simulink model "test_only"  (R2020a)
settings: Solver=FixedStepDiscrete  StartTime=0.0  StopTime=Parm_cnv_simulink_stopTime  FixedStep=Const_cnv_fundmt_stepSize  RelTol=1e-3  EnableMultiTasking=on
InitFcn:
  | preLoadFun
libraries: speedgoatlib_IO691 x9, canmsglib x9, MyLibrary x1, libtb_gen_canMsgCntr x1
Description:
  | - Add preLoadFun.m into Callbacks InitFcn
  | - Combine Sensata and Pirelle sensor inputs into one subsystem
  | - Two enumerators: defEnum_fun_tbm.m && def_vehFun_Enum.m
settings Model: SimulationMode=external  PauseTimes=49.73  NumberOfSteps=20  EnablePacing=on  PacingRate=112  Creator=jianjun.gao  LastModifiedBy=bowen.zheng
settings SolverCC: ConcurrentTasks=on  AlgebraicLoopSolver=LineSearch  AutoInsertRateTranBlk=on
settings DataIOCC: LimitDataPoints=on  SaveFormat=StructureWithTime  ReturnWorkspaceOutputs=off
settings OptimizationCC: BlockReduction=off  DefaultUnderspecifiedDataType=single  OptimizeBlockIOStorage=off  EnhancedBackFolding=on  PassReuseOutputArgsThreshold=0  ExpressionDepthLimit=2147483647  OptimizeBlockOrder=speed  DifferentSizesBufferReuse=on
settings DebuggingCC: UnderspecifiedInitializationDetection=Classic  MergeDetectMultiDrivingBlocksExec=none  SolverPrmCheckMsg=warning  ParameterTunabilityLossMsg=error  FcnCallInpInsideContextMsg=warning  BusObjectLabelMismatch=error  AllowSymbolicDim=off  StateNameClashWarn=warning  SFUnexpectedBacktrackingDiag=warning  SFNoUnconditionalDefaultTransitionDiag=warning  SFExecutionAtInitializationDiag=none  ArithmeticOperatorsInVariantConditions=warning
settings HardwareCC: ProdBitPerPointer=32  ProdBitPerSizeT=32  ProdBitPerPtrDiffT=32  ProdLargestAtomicFloat=None  ProdWordSize=32  ProdLongLongMode=on  ProdHWDeviceType=Generic->32-bit x86 compatible
settings ModelReferenceCC: PropagateSignalLabelsOutOfModel=off
settings SFSimCC: SimUseLocalCustomCode=off  MATLABDynamicMemAlloc=off  CustomCodeUndefinedFunction=UseInterfaceOnly
settings RTWCC: Description=Simulink Real-Time  SystemTargetFile=slrt.tlc  PackageName=addn_compled  TemplateMakefile=slrt_default_tmf  RTWUseLocalCustomCode=off  RTWUseSimCustomCode=on  BuildConfiguration=Faster Runs  CodeExecutionProfiling=on  RTWCompilerOptimization=on
settings CodeAppCC: ForceParamTrailComments=on  MaxIdLength=63  OperatorAnnotations=on
settings SimulinkRealTimeCC: SupportVariableSizeSignals=on  RL32LogTETModifier=off  xPCConcurrentTasks=on
settings ConfigComp: CovMetricSettings=dw  CovHtmlReporting=on  CovSaveCumulativeToWorkspaceVar=on  CovSaveSingleToWorkspaceVar=on  CovExternalEMLEnable=off
settings SimscapeCC: SimscapeNormalizeSystem=off
settings ConfigurationSet: Description=SimMechanics 2G

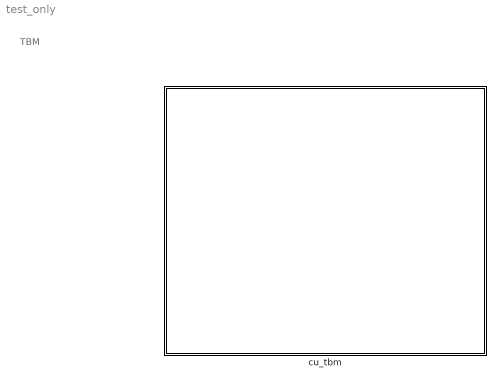
== system test_only ==
  note: TBM
  cu_tbm : Subsystem

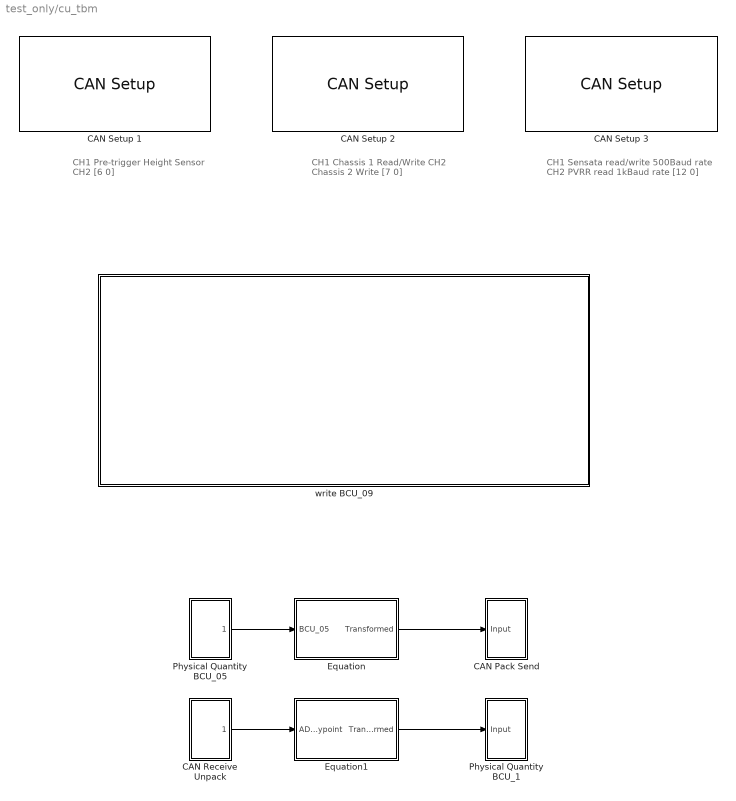
== system test_only/cu_tbm ==
  note: CH1 Pre-trigger Height Sensor
      | CH2
      | [6 0]
  note: CH1 Chassis 1 Read/Write
      | CH2 Chassis 2 Write
      | [7 0]
  note: CH1 Sensata read/write 500Baud rate
      | CH2 PVRR read 1kBaud rate
      | [12 0]
  CAN Pack Send : Subsystem
  CAN Receive Unpack : Subsystem
  CAN Setup 1 : speedgoatlib_IO691/CAN Setup   moduletype=IO691  id=1  pciSlot=[6 0]  chn1=CAN (HS)  chn2=CAN (HS)  chn3=Disabled  chn4=Disabled  initStruct=[]  termStruct=[]  ArbitrationbdrChn1=500 kBaud  ArbitrationManbdrChn1=[2,16,63,16]  FdbdrChn1=5.0 MBaud  FdManbdrChn1=[2,2,5,2]  ArbitrationbdrChn2=500 kBaud  ArbitrationManbdrChn2=[2,16,63,16]  FdbdrChn2=5.0 MBaud  FdManbdrChn2=[2,2,5,2]  ArbitrationbdrChn3=1.0 MBaud  ArbitrationManbdrChn3=[2,8,31,8]  FdbdrChn3=5.0 MBaud  FdManbdrChn3=[2,2,5,2]  ArbitrationbdrChn4=1.0 MBaud  ArbitrationManbdrChn4=[2,8,31,8]  FdbdrChn4=5.0 MBaud  FdManbdrChn4=[2,2,5,2]  moduleInitValues=[691 1 6 0]
      settings: SourceProductName=Simulink Real-Time: Speedgoat I/O Blockset
  CAN Setup 2 : speedgoatlib_IO691/CAN Setup   moduletype=IO691  id=2  pciSlot=[7 0]  chn1=CAN (HS)  chn2=CAN (HS)  chn3=Disabled  chn4=Disabled  initStruct=[]  termStruct=[]  ArbitrationbdrChn1=500 kBaud  ArbitrationManbdrChn1=[2,16,63,16]  FdbdrChn1=5.0 MBaud  FdManbdrChn1=[2,2,5,2]  ArbitrationbdrChn2=500 kBaud  ArbitrationManbdrChn2=[2,16,63,16]  FdbdrChn2=5.0 MBaud  FdManbdrChn2=[2,2,5,2]  ArbitrationbdrChn3=1.0 MBaud  ArbitrationManbdrChn3=[2,8,31,8]  FdbdrChn3=5.0 MBaud  FdManbdrChn3=[2,2,5,2]  ArbitrationbdrChn4=1.0 MBaud  ArbitrationManbdrChn4=[2,8,31,8]  FdbdrChn4=5.0 MBaud  FdManbdrChn4=[2,2,5,2]  moduleInitValues=[691 2 7 0]
      settings: SourceProductName=Simulink Real-Time: Speedgoat I/O Blockset
  CAN Setup 3 : speedgoatlib_IO691/CAN Setup   moduletype=IO691  id=4  pciSlot=[12 0]  chn1=CAN (HS)  chn2=CAN (HS)  chn3=Disabled  chn4=Disabled  initStruct=[]  termStruct=[]  ArbitrationbdrChn1=500 kBaud  ArbitrationManbdrChn1=[2,16,63,16]  FdbdrChn1=5.0 MBaud  FdManbdrChn1=[2,2,5,2]  ArbitrationbdrChn2=1.0 MBaud  ArbitrationManbdrChn2=[2,8,31,8]  FdbdrChn2=5.0 MBaud  FdManbdrChn2=[2,2,5,2]  ArbitrationbdrChn3=1.0 MBaud  ArbitrationManbdrChn3=[2,8,31,8]  FdbdrChn3=5.0 MBaud  FdManbdrChn3=[2,2,5,2]  ArbitrationbdrChn4=1.0 MBaud  ArbitrationManbdrChn4=[2,8,31,8]  FdbdrChn4=5.0 MBaud  FdManbdrChn4=[2,2,5,2]  moduleInitValues=[691 4 12 0]
      settings: SourceProductName=Simulink Real-Time: Speedgoat I/O Blockset
  Equation : Subsystem
  Equation1 : Subsystem
  Physical Quantity BCU_05 : Subsystem
  Physical Quantity BCU_1 : Subsystem
  write BCU_09 : Subsystem
  wires:
  Physical Quantity BCU_05/1(BCU_05) -> Equation/1(BCU_05)
  CAN Receive Unpack/1(Output) -> Equation1/1(ADC_Waypoint)
  Equation1/1(Transformed) -> Physical Quantity BCU_1/1(Input)
  Equation/1(Transformed) -> CAN Pack Send/1(Input)

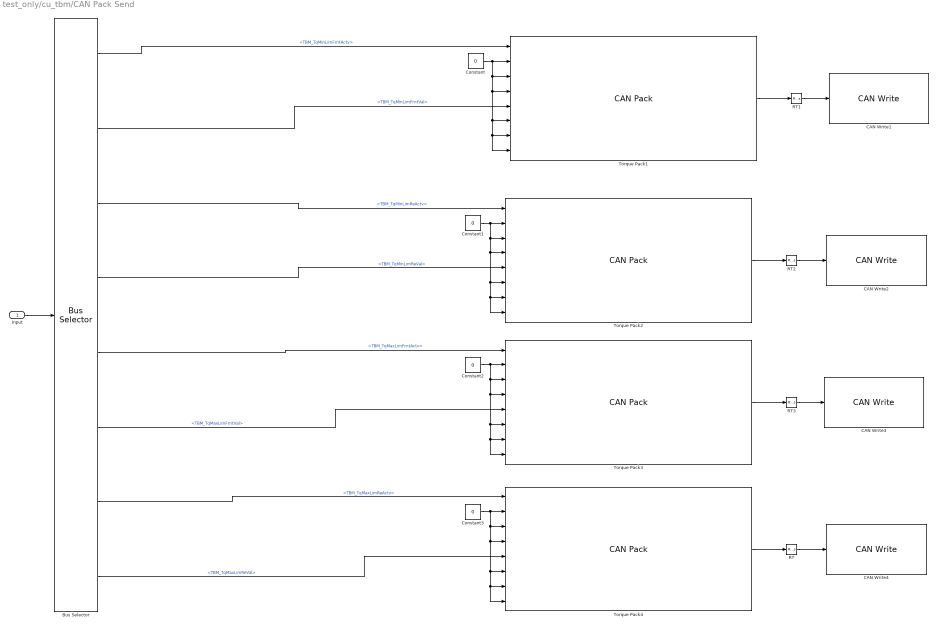
== system test_only/cu_tbm/CAN Pack Send ==
  Input : Inport
  Bus Selector : BusSelector  OutputSignals=TBM_TqMinLimFrntActv,TBM_TqMinLimFrntVal,TBM_TqMinLimReActv,TBM_TqMinLimReVal,TBM_TqMaxLimFrntActv,TBM_TqMaxLimFrntVal,TBM_TqMaxLimReActv,TBM_TqMaxLimReVal
  CAN Write{1..4} (4 alike) : speedgoatlib_IO691/CAN Write  id=2  ts=0.02  channel=1  messageType=CAN  enableStatusPort=off  canType=CAN (HS)  initValues=[691 2 0.02 0 1 1 0]
      settings: SourceProductName=Simulink Real-Time: Speedgoat I/O Blockset
  Constant{,1..3} (4 alike) : Constant  Value=0  OutDataTypeStr=single
  RT{,1..3} (4 alike) : RateTransition  OutPortSampleTime=0.02
  Torque Pack1 : canmsglib/CAN Pack  CANdbFile=.\support\dbc\NIO_NT2_Chassis2_CAN_Official_Release_V_1_1_DA_02.dbc  MsgList=ADC1_WayPoint01  MsgName=ADC1_WayPoint01  MsgIDType=Standard (11-bit identifier)  MsgIdentifier=214  MsgLength=8  Remote=off  ApplyMinMax=off  BusOutput=off  SignalInfo={'LD_Confidence_1','24','4','BE','unsigned','Standard','0','0.1','0','0','1.5';'LD_First_End_1','51','7','BE','unsigned','Standard','0','1','0','0','127';'LD_First_Start_1','16','8','BE','unsigned','Standard','0','0.1','0','0','25.5';'LD_First_Type_1','28','4','BE','unsigned','Standard','0','1','0','0','15';'LD_Line_First_C0_1','56','11','BE','unsigned','Standard','0','0.01','-10.24','-10.24','10.23';'LD_Line_First_C1_1','43','13','BE','unsigned','Standard','0','0.0001','-0.4096','-0.4096','0.4095';'LD_Line_First_C2_1','0','8','BE','unsigned','Standard','0','0.0001','-0.0128','-0.0128','0.0127';'LD_Line_First_C3_1','8','8','BE','unsigned','Standard','0','1e-06','-0.000128','-0.000128','0.000127'}
      settings: SourceProductBaseCode=ME,VN  DataFormat=CANdb specified signals
  Torque Pack2 : canmsglib/CAN Pack  CANdbFile=.\support\dbc\NIO_NT2_Chassis2_CAN_Official_Release_V_1_1_DA_02.dbc  MsgList=ADC1_WayPoint02  MsgName=ADC1_WayPoint02  MsgIDType=Standard (11-bit identifier)  MsgIdentifier=215  MsgLength=8  Remote=off  ApplyMinMax=off  BusOutput=off  SignalInfo={'LD_Confidence_2','24','4','BE','unsigned','Standard','0','0.1','0','0','1.5';'LD_First_End_2','51','7','BE','unsigned','Standard','0','1','0','0','127';'LD_First_Start_2','16','8','BE','unsigned','Standard','0','0.1','0','0','25.5';'LD_First_Type_2','28','4','BE','unsigned','Standard','0','1','0','0','15';'LD_Line_First_C0_2','56','11','BE','unsigned','Standard','0','0.01','-10.24','-10.24','10.23';'LD_Line_First_C1_2','43','13','BE','unsigned','Standard','0','0.0001','-0.4096','-0.4096','0.4095';'LD_Line_First_C2_2','0','8','BE','unsigned','Standard','0','0.0001','-0.0128','-0.0128','0.0127';'LD_Line_First_C3_2','8','8','BE','unsigned','Standard','0','1e-06','-0.000128','-0.000128','0.000127'}
      settings: SourceProductBaseCode=ME,VN  DataFormat=CANdb specified signals
  Torque Pack3 : canmsglib/CAN Pack  CANdbFile=.\support\dbc\NIO_NT2_Chassis2_CAN_Official_Release_V_1_1_DA_02.dbc  MsgList=ADC1_WayPoint03  MsgName=ADC1_WayPoint03  MsgIDType=Standard (11-bit identifier)  MsgIdentifier=216  MsgLength=8  Remote=off  ApplyMinMax=off  BusOutput=off  SignalInfo={'LD_Confidence_3','24','4','BE','unsigned','Standard','0','0.1','0','0','1.5';'LD_First_End_3','51','7','BE','unsigned','Standard','0','1','0','0','127';'LD_First_Start_3','16','8','BE','unsigned','Standard','0','0.1','0','0','25.5';'LD_First_Type_3','28','4','BE','unsigned','Standard','0','1','0','0','15';'LD_Line_First_C0_3','56','11','BE','unsigned','Standard','0','0.01','-10.24','-10.24','10.23';'LD_Line_First_C1_3','43','13','BE','unsigned','Standard','0','0.0001','-0.4096','-0.4096','0.4095';'LD_Line_First_C2_3','0','8','BE','unsigned','Standard','0','0.0001','-0.0128','-0.0128','0.0127';'LD_Line_First_C3_3','8','8','BE','unsigned','Standard','0','1e-06','-0.000128','-0.000128','0.000127'}
      settings: SourceProductBaseCode=ME,VN  DataFormat=CANdb specified signals
  Torque Pack4 : canmsglib/CAN Pack  CANdbFile=.\support\dbc\NIO_NT2_Chassis2_CAN_Official_Release_V_1_1_DA_02.dbc  MsgList=ADC1_WayPoint04  MsgName=ADC1_WayPoint04  MsgIDType=Standard (11-bit identifier)  MsgIdentifier=217  MsgLength=8  Remote=off  ApplyMinMax=off  BusOutput=off  SignalInfo={'LD_Confidence_4','24','4','BE','unsigned','Standard','0','0.1','0','0','1.5';'LD_First_End_4','51','7','BE','unsigned','Standard','0','1','0','0','127';'LD_First_Start_4','16','8','BE','unsigned','Standard','0','0.1','0','0','25.5';'LD_First_Type_4','28','4','BE','unsigned','Standard','0','1','0','0','15';'LD_Line_First_C0_4','56','11','BE','unsigned','Standard','0','0.01','-10.24','-10.24','10.23';'LD_Line_First_C1_4','43','13','BE','unsigned','Standard','0','0.0001','-0.4096','-0.4096','0.4095';'LD_Line_First_C2_4','0','8','BE','unsigned','Standard','0','0.0001','-0.0128','-0.0128','0.0127';'LD_Line_First_C3_4','8','8','BE','unsigned','Standard','0','1e-06','-0.000128','-0.000128','0.000127'}
      settings: SourceProductBaseCode=ME,VN  DataFormat=CANdb specified signals
  wires:
  RT/1 -> CAN Write4/1
  RT3/1 -> CAN Write3/1
  Torque Pack3/1 -> RT3/1
  Torque Pack4/1 -> RT/1
  Torque Pack2/1 -> RT2/1
  RT2/1 -> CAN Write2/1
  Input/1 -> Bus Selector/1
  Bus Selector/1 -> Torque Pack1/1  "<TBM_TqMinLimFrntActv>"
  RT1/1 -> CAN Write1/1
  Torque Pack1/1 -> RT1/1
  Bus Selector/2 -> Torque Pack1/5  "<TBM_TqMinLimFrntVal>"
  Bus Selector/3 -> Torque Pack2/1  "<TBM_TqMinLimReActv>"
  Bus Selector/4 -> Torque Pack2/5  "<TBM_TqMinLimReVal>"
  Bus Selector/5 -> Torque Pack3/1  "<TBM_TqMaxLimFrntActv>"
  Bus Selector/6 -> Torque Pack3/5  "<TBM_TqMaxLimFrntVal>"
  Bus Selector/7 -> Torque Pack4/1  "<TBM_TqMaxLimReActv>"
  Bus Selector/8 -> Torque Pack4/5  "<TBM_TqMaxLimReVal>"
  Constant/1 -> Torque Pack1/8, Torque Pack1/7, Torque Pack1/6, Torque Pack1/4, Torque Pack1/3, Torque Pack1/2
  Constant1/1 -> Torque Pack2/2, Torque Pack2/3, Torque Pack2/4, Torque Pack2/6, Torque Pack2/8, Torque Pack2/7
  Constant2/1 -> Torque Pack3/2, Torque Pack3/3, Torque Pack3/4, Torque Pack3/6, Torque Pack3/7, Torque Pack3/8
  Constant3/1 -> Torque Pack4/2, Torque Pack4/3, Torque Pack4/4, Torque Pack4/6, Torque Pack4/8, Torque Pack4/7

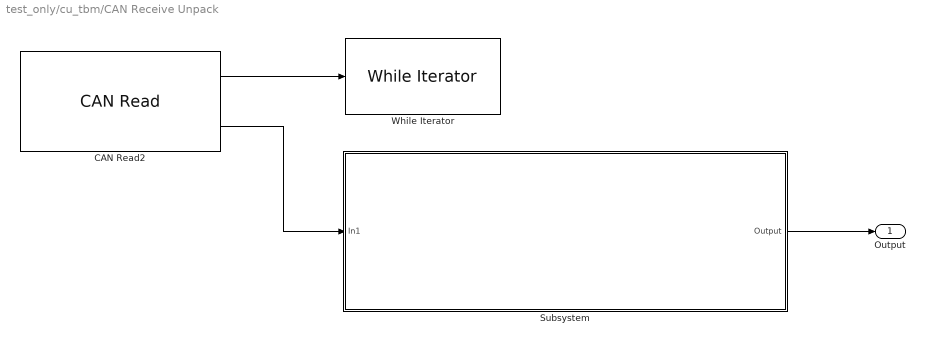
== system test_only/cu_tbm/CAN Receive Unpack ==
  CAN Read2 : speedgoatlib_IO691/CAN Read  id=2  ts=-1  channel=2  messageType=CAN  canType=CAN (HS)  initValues=[691 2 -1 1 1 1]
      settings: SourceProductName=Simulink Real-Time: Speedgoat I/O Blockset
  Subsystem : Subsystem
  While Iterator : WhileIterator  MaxIters=-1  WhileBlockType=do-while
  Output : Outport
  wires:
  CAN Read2/2 -> Subsystem/1(In1)
  CAN Read2/1 -> While Iterator/1
  Subsystem/1(Output) -> Output/1

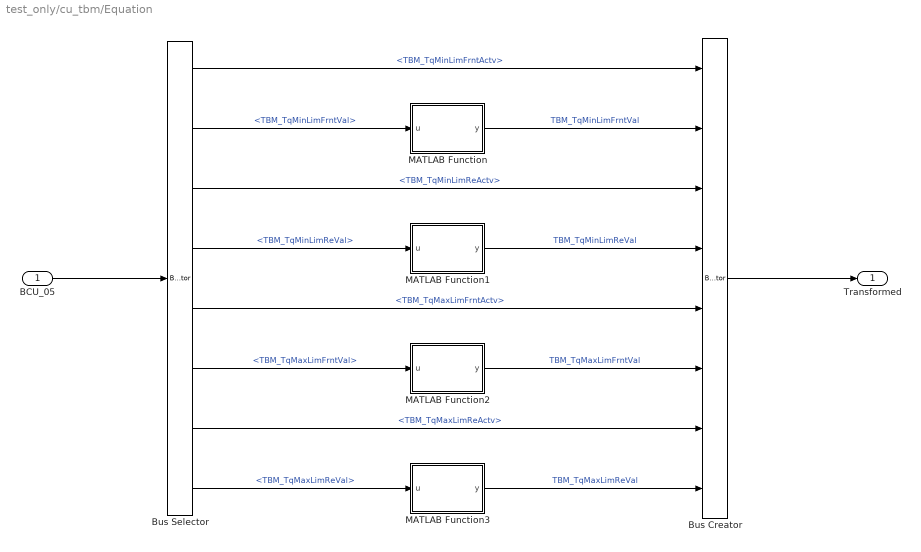
== system test_only/cu_tbm/Equation ==
  BCU_05 : Inport
  Bus Creator : BusCreator  Inputs=8
  Bus Selector : BusSelector  OutputSignals=TBM_TqMinLimFrntActv,TBM_TqMinLimFrntVal,TBM_TqMinLimReActv,TBM_TqMinLimReVal,TBM_TqMaxLimFrntActv,TBM_TqMaxLimFrntVal,TBM_TqMaxLimReActv,TBM_TqMaxLimReVal
  MATLAB Function : MATLAB Function  TreatAsAtomicUnit=on
  MATLAB Function1 : MATLAB Function  TreatAsAtomicUnit=on
  MATLAB Function2 : MATLAB Function  TreatAsAtomicUnit=on
  MATLAB Function3 : MATLAB Function  TreatAsAtomicUnit=on
  Transformed : Outport
  wires:
  BCU_05/1 -> Bus Selector/1
  Bus Creator/1 -> Transformed/1
  Bus Selector/1 -> Bus Creator/1  "<TBM_TqMinLimFrntActv>"
  Bus Selector/3 -> Bus Creator/3  "<TBM_TqMinLimReActv>"
  Bus Selector/5 -> Bus Creator/5  "<TBM_TqMaxLimFrntActv>"
  Bus Selector/7 -> Bus Creator/7  "<TBM_TqMaxLimReActv>"
  Bus Selector/2 -> MATLAB Function/1(u)  "<TBM_TqMinLimFrntVal>"
  MATLAB Function/1(y) -> Bus Creator/2  "TBM_TqMinLimFrntVal"
  Bus Selector/8 -> MATLAB Function3/1(u)  "<TBM_TqMaxLimReVal>"
  Bus Selector/6 -> MATLAB Function2/1(u)  "<TBM_TqMaxLimFrntVal>"
  Bus Selector/4 -> MATLAB Function1/1(u)  "<TBM_TqMinLimReVal>"
  MATLAB Function1/1(y) -> Bus Creator/4  "TBM_TqMinLimReVal"
  MATLAB Function2/1(y) -> Bus Creator/6  "TBM_TqMaxLimFrntVal"
  MATLAB Function3/1(y) -> Bus Creator/8  "TBM_TqMaxLimReVal"

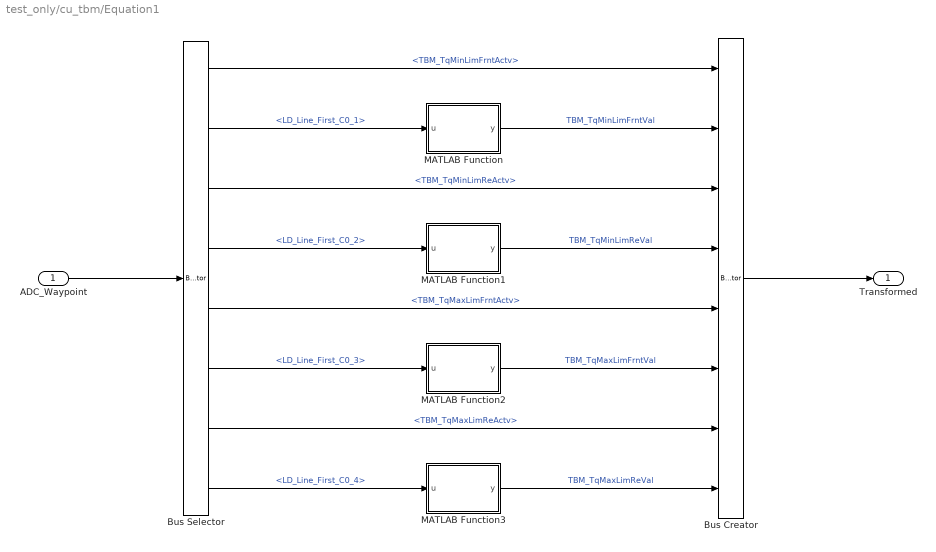
== system test_only/cu_tbm/Equation1 ==
  ADC_Waypoint : Inport
  Bus Creator : BusCreator  Inputs=8
  Bus Selector : BusSelector  OutputSignals=TBM_TqMinLimFrntActv,LD_Line_First_C0_1,TBM_TqMinLimReActv,LD_Line_First_C0_2,TBM_TqMaxLimFrntActv,LD_Line_First_C0_3,TBM_TqMaxLimReActv,LD_Line_First_C0_4
  MATLAB Function : MATLAB Function  TreatAsAtomicUnit=on
  MATLAB Function1 : MATLAB Function  TreatAsAtomicUnit=on
  MATLAB Function2 : MATLAB Function  TreatAsAtomicUnit=on
  MATLAB Function3 : MATLAB Function  TreatAsAtomicUnit=on
  Transformed : Outport
  wires:
  ADC_Waypoint/1 -> Bus Selector/1
  Bus Creator/1 -> Transformed/1
  Bus Selector/1 -> Bus Creator/1  "<TBM_TqMinLimFrntActv>"
  Bus Selector/3 -> Bus Creator/3  "<TBM_TqMinLimReActv>"
  Bus Selector/5 -> Bus Creator/5  "<TBM_TqMaxLimFrntActv>"
  Bus Selector/7 -> Bus Creator/7  "<TBM_TqMaxLimReActv>"
  Bus Selector/2 -> MATLAB Function/1(u)  "<LD_Line_First_C0_1>"
  MATLAB Function/1(y) -> Bus Creator/2  "TBM_TqMinLimFrntVal"
  Bus Selector/8 -> MATLAB Function3/1(u)  "<LD_Line_First_C0_4>"
  Bus Selector/6 -> MATLAB Function2/1(u)  "<LD_Line_First_C0_3>"
  Bus Selector/4 -> MATLAB Function1/1(u)  "<LD_Line_First_C0_2>"
  MATLAB Function1/1(y) -> Bus Creator/4  "TBM_TqMinLimReVal"
  MATLAB Function2/1(y) -> Bus Creator/6  "TBM_TqMaxLimFrntVal"
  MATLAB Function3/1(y) -> Bus Creator/8  "TBM_TqMaxLimReVal"

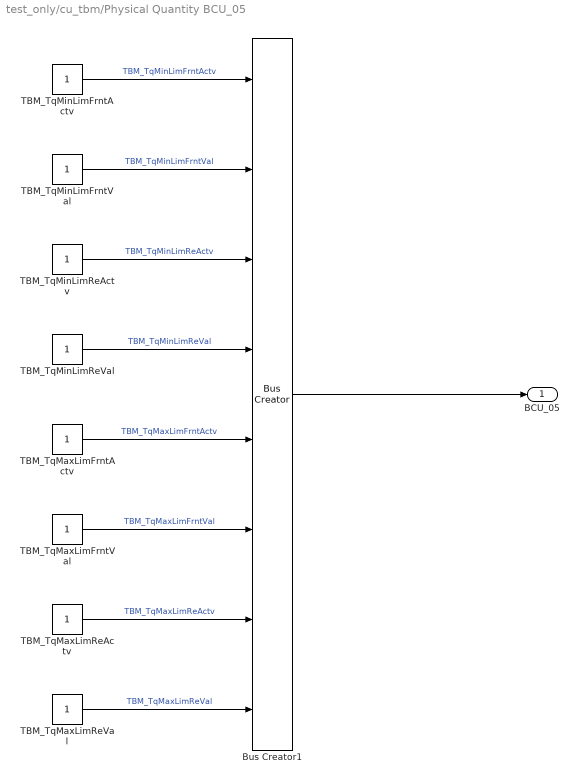
== system test_only/cu_tbm/Physical Quantity BCU_05 ==
  Bus Creator1 : BusCreator  Inputs=8
  TBM_TqMaxLimFrntActv : Constant  OutDataTypeStr=single
  TBM_TqMaxLimFrntVal : Constant  OutDataTypeStr=single
  TBM_TqMaxLimReActv : Constant  OutDataTypeStr=single
  TBM_TqMaxLimReVal : Constant  OutDataTypeStr=single
  TBM_TqMinLimFrntActv : Constant  OutDataTypeStr=single
  TBM_TqMinLimFrntVal : Constant  OutDataTypeStr=single
  TBM_TqMinLimReActv : Constant  OutDataTypeStr=single
  TBM_TqMinLimReVal : Constant  OutDataTypeStr=single
  BCU_05 : Outport  OutDataTypeStr=single  PortDimensions=8
  wires:
  TBM_TqMaxLimReVal/1 -> Bus Creator1/8  "TBM_TqMaxLimReVal"
  Bus Creator1/1 -> BCU_05/1
  TBM_TqMinLimFrntVal/1 -> Bus Creator1/2  "TBM_TqMinLimFrntVal"
  TBM_TqMinLimReVal/1 -> Bus Creator1/4  "TBM_TqMinLimReVal"
  TBM_TqMinLimReActv/1 -> Bus Creator1/3  "TBM_TqMinLimReActv"
  TBM_TqMaxLimFrntActv/1 -> Bus Creator1/5  "TBM_TqMaxLimFrntActv"
  TBM_TqMaxLimReActv/1 -> Bus Creator1/7  "TBM_TqMaxLimReActv"
  TBM_TqMinLimFrntActv/1 -> Bus Creator1/1  "TBM_TqMinLimFrntActv"
  TBM_TqMaxLimFrntVal/1 -> Bus Creator1/6  "TBM_TqMaxLimFrntVal"

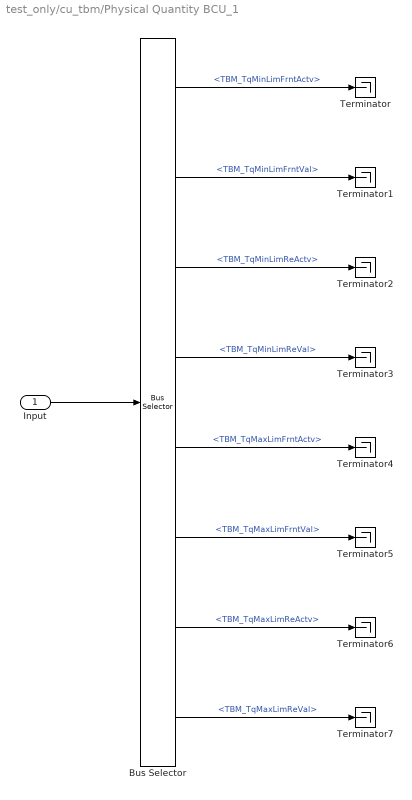
== system test_only/cu_tbm/Physical Quantity BCU_1 ==
  Input : Inport
  Bus Selector : BusSelector  OutputSignals=TBM_TqMinLimFrntActv,TBM_TqMinLimFrntVal,TBM_TqMinLimReActv,TBM_TqMinLimReVal,TBM_TqMaxLimFrntActv,TBM_TqMaxLimFrntVal,TBM_TqMaxLimReActv,TBM_TqMaxLimReVal
  Terminator{,1..7} (8 alike) : Terminator
  wires:
  Bus Selector/8 -> Terminator7/1  "<TBM_TqMaxLimReVal>"
  Bus Selector/2 -> Terminator1/1  "<TBM_TqMinLimFrntVal>"
  Bus Selector/4 -> Terminator3/1  "<TBM_TqMinLimReVal>"
  Bus Selector/3 -> Terminator2/1  "<TBM_TqMinLimReActv>"
  Bus Selector/5 -> Terminator4/1  "<TBM_TqMaxLimFrntActv>"
  Bus Selector/7 -> Terminator6/1  "<TBM_TqMaxLimReActv>"
  Bus Selector/1 -> Terminator/1  "<TBM_TqMinLimFrntActv>"
  Bus Selector/6 -> Terminator5/1  "<TBM_TqMaxLimFrntVal>"
  Input/1 -> Bus Selector/1

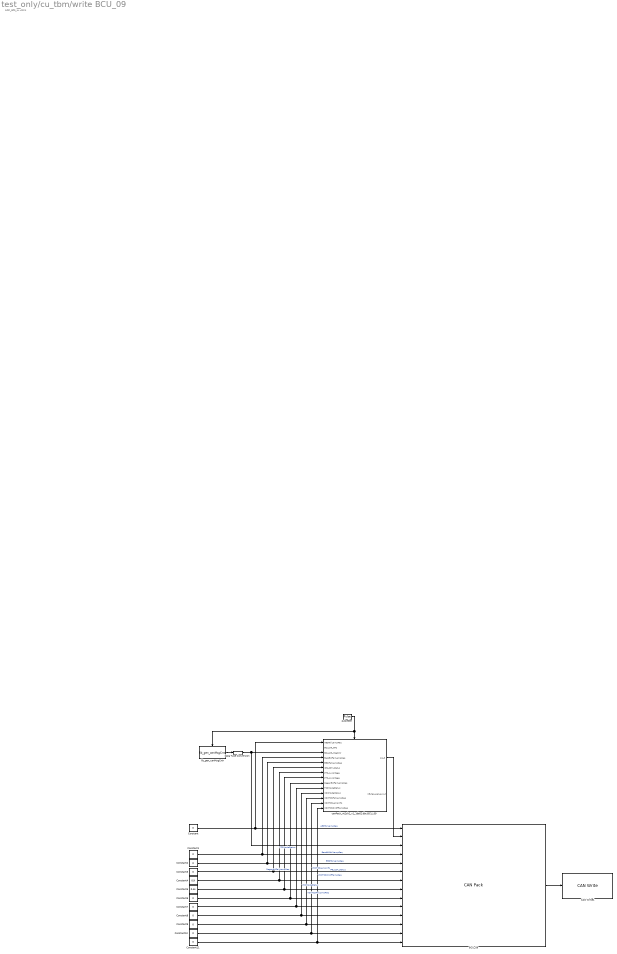
== system test_only/cu_tbm/write BCU_09 ==
  note: ADC_EPS_01 20ms
  BCU_09 : canmsglib/CAN Pack  CANdbFile=C:\Users\bowen.zheng\Desktop\spdGoat_prj_20230315\spdGoat_prj_20230315\support\dbc\NIO_NT2_Chassis2_CAN_Official_Release_V_1_1_DA_02.dbc  MsgList=(none)  MsgName=BCU_09  MsgIDType=Standard (11-bit identifier)  MsgIdentifier=591  MsgLength=8  Remote=off  ApplyMinMax=off  BusOutput=off  SignalInfo={'ABSFailLampReq','37','1','BE','unsigned','Standard','0','1','0','0','1';'BCU_09_CRC','0','8','BE','unsigned','Standard','0','1','0','0','255';'BCU_09_MsgCntr','12','4','BE','unsigned','Standard','0','1','0','0','15';'BascBrkFailLampReq','32','2','BE','unsigned','Standard','0','1','0','0','3';'EBDFailLampReq','34','1','BE','unsigned','Standard','0','1','0','0','1';'IPB_CST_Status','38','2','BE','unsigned','Standard','0','1','0','0','3';'PTS_1_Voltage','17','9','BE','unsigned','Standard','0','0.01','-0.5','-0.5','4.61';'PTS_2_Voltage','24','9','BE','unsigned','Standard','0','0.01','-0.5','-0.5','4.61';'RegenBrkFailLampReq','10','1','BE','unsigned','Standard','0','1','0','0','1';'TCSModeStatus','45','3','BE','unsigned','Standard','0','1','0','0','7';'VDCModeStatus','42','3','BE','unsigned','Standard','0','1','0','0','7';'VDCTCSFailLampReq','36','1','BE','unsigned','Standard','0','1','0','0','1';'VDCTCSLampInfo','35','1','BE','unsigned','Standard','0','1','0','0','1';'VDCTCSOnOfflampReq','11','1','BE','unsigned','Standard','0','1','0','0','1'}
      settings: SourceProductBaseCode=ME,VN  DataFormat=CANdb specified signals
  CAN Write1 : speedgoatlib_IO691/CAN Write  id=2  ts=0.1  channel=2  messageType=CAN  enableStatusPort=off  canType=CAN (HS)  initValues=[691 2 0.1 1 1 1 0]
      settings: SourceProductName=Simulink Real-Time: Speedgoat I/O Blockset
  Constant{,1..3,6..11} (10 alike) : Constant  Value=0  OutDataTypeStr=single
  Constant4 : Constant  Value=0.9  OutDataTypeStr=single
  Constant5 : Constant  Value=0.44  OutDataTypeStr=single
  Data Type Conversion : DataTypeConversion  OutDataTypeStr=single  RndMeth=Nearest
  canPack_nt2ch2_v1_1da02.dbc:BCU_09 : Subsystem
  lib_gen_canMsgCntr : libtb_gen_canMsgCntr/lib_gen_canMsgCntr  SystemSampleTime=-1  Latency=0  AutoFrameSizeCalculation=off
  pulseGen : DiscretePulseGenerator  PulseType=Time based  Period=0.1  PulseWidth=50
  wires:
  BCU_09/1 -> CAN Write1/1
  lib_gen_canMsgCntr/1 -> Data Type Conversion/1
  Constant/1 -> canPack_nt2ch2_v1_1da02.dbc:BCU_09/1(ABSFailLampReq), BCU_09/1  "ABSFailLampReq"
  Constant1/1 -> canPack_nt2ch2_v1_1da02.dbc:BCU_09/4(BascBrkFailLampReq), BCU_09/4  "BascBrkFailLampReq"
  Constant2/1 -> canPack_nt2ch2_v1_1da02.dbc:BCU_09/5(EBDFailLampReq), BCU_09/5  "EBDFailLampReq"
  Constant3/1 -> canPack_nt2ch2_v1_1da02.dbc:BCU_09/6(IPB_CST_Status), BCU_09/6  "IPB_CST_Status"
  Constant4/1 -> canPack_nt2ch2_v1_1da02.dbc:BCU_09/7(PTS_1_Voltage), BCU_09/7
  Constant5/1 -> canPack_nt2ch2_v1_1da02.dbc:BCU_09/8(PTS_2_Voltage), BCU_09/8
  Constant6/1 -> canPack_nt2ch2_v1_1da02.dbc:BCU_09/9(RegenBrkFailLampReq), BCU_09/9  "RegenBrkFailLampReq"
  Constant7/1 -> canPack_nt2ch2_v1_1da02.dbc:BCU_09/10(TCSModeStatus), BCU_09/10  "TCSModeStatus"
  Constant8/1 -> canPack_nt2ch2_v1_1da02.dbc:BCU_09/11(VDCModeStatus), BCU_09/11  "VDCModeStatus"
  Constant9/1 -> BCU_09/12, canPack_nt2ch2_v1_1da02.dbc:BCU_09/12(VDCTCSFailLampReq)  "VDCTCSFailLampReq"
  Constant10/1 -> canPack_nt2ch2_v1_1da02.dbc:BCU_09/13(VDCTCSLampInfo), BCU_09/13  "VDCTCSLampInfo"
  Constant11/1 -> canPack_nt2ch2_v1_1da02.dbc:BCU_09/14(VDCTCSOnOfflampReq), BCU_09/14  "VDCTCSOnOfflampReq"
  pulseGen/1 -> lib_gen_canMsgCntr/Trigger, canPack_nt2ch2_v1_1da02.dbc:BCU_09/Trigger
  Data Type Conversion/1 -> BCU_09/3, canPack_nt2ch2_v1_1da02.dbc:BCU_09/3(BCU_09_MsgCntr)
  canPack_nt2ch2_v1_1da02.dbc:BCU_09/1(crc_8) -> BCU_09/2

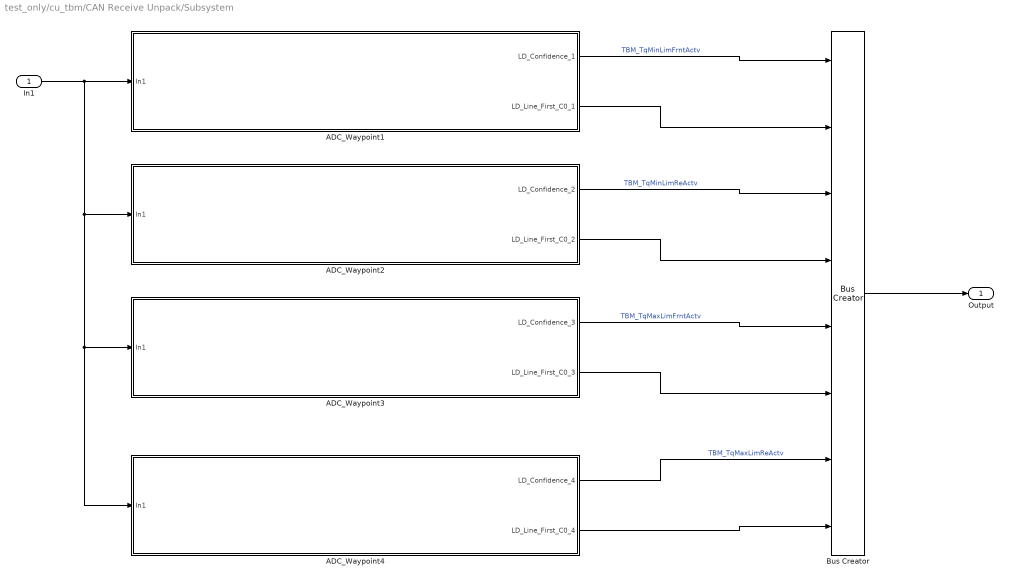
== system test_only/cu_tbm/CAN Receive Unpack/Subsystem ==
  In1 : Inport
  ADC_Waypoint1 : Subsystem
  ADC_Waypoint2 : Subsystem
  ADC_Waypoint3 : Subsystem
  ADC_Waypoint4 : Subsystem
  Bus Creator : BusCreator  Inputs=8
  Output : Outport
  wires:
  In1/1 -> ADC_Waypoint4/1(In1), ADC_Waypoint3/1(In1), ADC_Waypoint2/1(In1), ADC_Waypoint1/1(In1)
  ADC_Waypoint1/1(LD_Confidence_1) -> Bus Creator/1  "TBM_TqMinLimFrntActv"
  ADC_Waypoint1/2(LD_Line_First_C0_1) -> Bus Creator/2
  ADC_Waypoint2/1(LD_Confidence_2) -> Bus Creator/3  "TBM_TqMinLimReActv"
  ADC_Waypoint2/2(LD_Line_First_C0_2) -> Bus Creator/4
  ADC_Waypoint3/1(LD_Confidence_3) -> Bus Creator/5  "TBM_TqMaxLimFrntActv"
  ADC_Waypoint3/2(LD_Line_First_C0_3) -> Bus Creator/6
  ADC_Waypoint4/1(LD_Confidence_4) -> Bus Creator/7  "TBM_TqMaxLimReActv"
  ADC_Waypoint4/2(LD_Line_First_C0_4) -> Bus Creator/8
  Bus Creator/1 -> Output/1

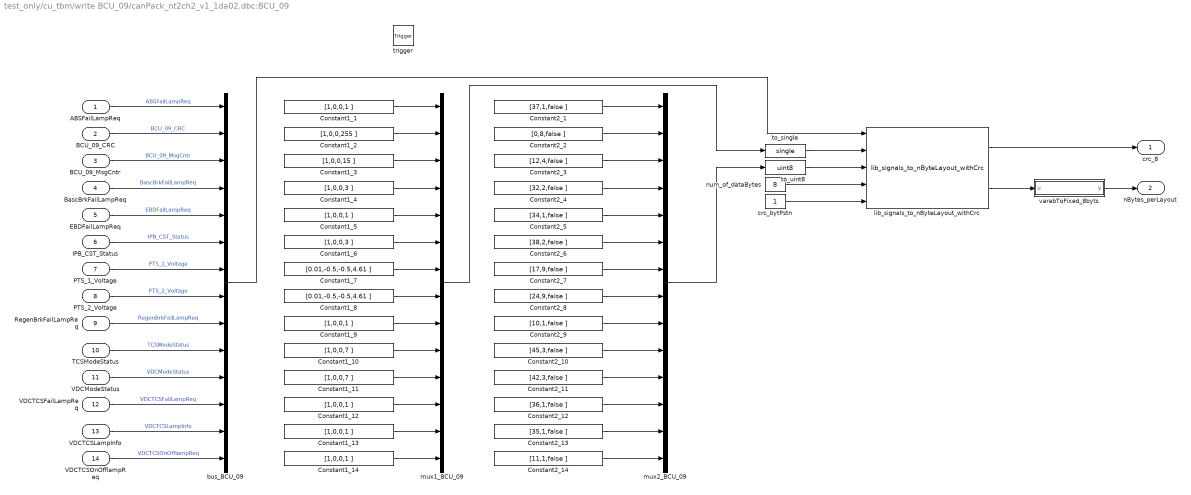
== system test_only/cu_tbm/write BCU_09/canPack_nt2ch2_v1_1da02.dbc:BCU_09 ==
  ABSFailLampReq : Inport
  BCU_09_CRC : Inport  Port=2
  BCU_09_MsgCntr : Inport  Port=3
  BascBrkFailLampReq : Inport  Port=4
  EBDFailLampReq : Inport  Port=5
  IPB_CST_Status : Inport  Port=6
  PTS_1_Voltage : Inport  Port=7
  PTS_2_Voltage : Inport  Port=8
  RegenBrkFailLampReq : Inport  Port=9
  TCSModeStatus : Inport  Port=10
  VDCModeStatus : Inport  Port=11
  VDCTCSFailLampReq : Inport  Port=12
  VDCTCSLampInfo : Inport  Port=13
  VDCTCSOnOfflampReq : Inport  Port=14
  trigger : TriggerPort  TriggerType=either  VariantControl=Variant  PortDimensions=1
  Constant1_{1,5,9,12..14} (6 alike) : Constant  Value=[1,0,0,1 ]  SampleTime=-1
  Constant1_10 : Constant  Value=[1,0,0,7 ]  SampleTime=-1
  Constant1_11 : Constant  Value=[1,0,0,7 ]  SampleTime=-1
  Constant1_2 : Constant  Value=[1,0,0,255 ]  SampleTime=-1
  Constant1_3 : Constant  Value=[1,0,0,15 ]  SampleTime=-1
  Constant1_4 : Constant  Value=[1,0,0,3 ]  SampleTime=-1
  Constant1_6 : Constant  Value=[1,0,0,3 ]  SampleTime=-1
  Constant1_7 : Constant  Value=[0.01,-0.5,-0.5,4.61 ]  SampleTime=-1
  Constant1_8 : Constant  Value=[0.01,-0.5,-0.5,4.61 ]  SampleTime=-1
  Constant2_1 : Constant  Value=[37,1,false ]  SampleTime=-1
  Constant2_10 : Constant  Value=[45,3,false ]  SampleTime=-1
  Constant2_11 : Constant  Value=[42,3,false ]  SampleTime=-1
  Constant2_12 : Constant  Value=[36,1,false ]  SampleTime=-1
  Constant2_13 : Constant  Value=[35,1,false ]  SampleTime=-1
  Constant2_14 : Constant  Value=[11,1,false ]  SampleTime=-1
  Constant2_2 : Constant  Value=[0,8,false ]  SampleTime=-1
  Constant2_3 : Constant  Value=[12,4,false ]  SampleTime=-1
  Constant2_4 : Constant  Value=[32,2,false ]  SampleTime=-1
  Constant2_5 : Constant  Value=[34,1,false ]  SampleTime=-1
  Constant2_6 : Constant  Value=[38,2,false ]  SampleTime=-1
  Constant2_7 : Constant  Value=[17,9,false ]  SampleTime=-1
  Constant2_8 : Constant  Value=[24,9,false ]  SampleTime=-1
  Constant2_9 : Constant  Value=[10,1,false ]  SampleTime=-1
  bus_BCU_09 : BusCreator  Inputs=14
  crc_bytPstn : Constant  OutDataTypeStr=uint8  SampleTime=-1
  lib_signals_to_nByteLayout_withCrc : MyLibrary/lib_signals_to_nByteLayout_withCrc  SystemSampleTime=-1  Latency=0  AutoFrameSizeCalculation=off
  mux1_BCU_09 : Mux  Inputs=14
  mux2_BCU_09 : Mux  Inputs=14
  num_of_dataBytes : Constant  Value=8  OutDataTypeStr=uint8  SampleTime=-1
  to_single : DataTypeConversion  OutDataTypeStr=single
  to_uint8 : DataTypeConversion  OutDataTypeStr=uint8
  varabToFixed_8byts : MATLAB Function  TreatAsAtomicUnit=on
  crc_8 : Outport
  nBytes_perLayout : Outport  Port=2
  wires:
  ABSFailLampReq/1 -> bus_BCU_09/1  "ABSFailLampReq"
  BCU_09_CRC/1 -> bus_BCU_09/2  "BCU_09_CRC"
  BCU_09_MsgCntr/1 -> bus_BCU_09/3  "BCU_09_MsgCntr"
  BascBrkFailLampReq/1 -> bus_BCU_09/4  "BascBrkFailLampReq"
  EBDFailLampReq/1 -> bus_BCU_09/5  "EBDFailLampReq"
  IPB_CST_Status/1 -> bus_BCU_09/6  "IPB_CST_Status"
  PTS_1_Voltage/1 -> bus_BCU_09/7  "PTS_1_Voltage"
  PTS_2_Voltage/1 -> bus_BCU_09/8  "PTS_2_Voltage"
  RegenBrkFailLampReq/1 -> bus_BCU_09/9  "RegenBrkFailLampReq"
  TCSModeStatus/1 -> bus_BCU_09/10  "TCSModeStatus"
  VDCModeStatus/1 -> bus_BCU_09/11  "VDCModeStatus"
  VDCTCSFailLampReq/1 -> bus_BCU_09/12  "VDCTCSFailLampReq"
  VDCTCSLampInfo/1 -> bus_BCU_09/13  "VDCTCSLampInfo"
  VDCTCSOnOfflampReq/1 -> bus_BCU_09/14  "VDCTCSOnOfflampReq"
  Constant1_1/1 -> mux1_BCU_09/1
  Constant2_1/1 -> mux2_BCU_09/1
  Constant1_2/1 -> mux1_BCU_09/2
  Constant2_2/1 -> mux2_BCU_09/2
  Constant1_3/1 -> mux1_BCU_09/3
  Constant2_3/1 -> mux2_BCU_09/3
  Constant1_4/1 -> mux1_BCU_09/4
  Constant2_4/1 -> mux2_BCU_09/4
  Constant1_5/1 -> mux1_BCU_09/5
  Constant2_5/1 -> mux2_BCU_09/5
  Constant1_6/1 -> mux1_BCU_09/6
  Constant2_6/1 -> mux2_BCU_09/6
  Constant1_7/1 -> mux1_BCU_09/7
  Constant2_7/1 -> mux2_BCU_09/7
  Constant1_8/1 -> mux1_BCU_09/8
  Constant2_8/1 -> mux2_BCU_09/8
  Constant1_9/1 -> mux1_BCU_09/9
  Constant2_9/1 -> mux2_BCU_09/9
  Constant1_10/1 -> mux1_BCU_09/10
  Constant2_10/1 -> mux2_BCU_09/10
  Constant1_11/1 -> mux1_BCU_09/11
  Constant2_11/1 -> mux2_BCU_09/11
  Constant1_12/1 -> mux1_BCU_09/12
  Constant2_12/1 -> mux2_BCU_09/12
  Constant1_13/1 -> mux1_BCU_09/13
  Constant2_13/1 -> mux2_BCU_09/13
  Constant1_14/1 -> mux1_BCU_09/14
  Constant2_14/1 -> mux2_BCU_09/14
  bus_BCU_09/1 -> lib_signals_to_nByteLayout_withCrc/1
  mux1_BCU_09/1 -> to_single/1
  to_single/1 -> lib_signals_to_nByteLayout_withCrc/2
  mux2_BCU_09/1 -> to_uint8/1
  to_uint8/1 -> lib_signals_to_nByteLayout_withCrc/3
  lib_signals_to_nByteLayout_withCrc/1 -> crc_8/1
  num_of_dataBytes/1 -> lib_signals_to_nByteLayout_withCrc/4
  lib_signals_to_nByteLayout_withCrc/2 -> varabToFixed_8byts/1(u)
  varabToFixed_8byts/1(y) -> nBytes_perLayout/1
  crc_bytPstn/1 -> lib_signals_to_nByteLayout_withCrc/5

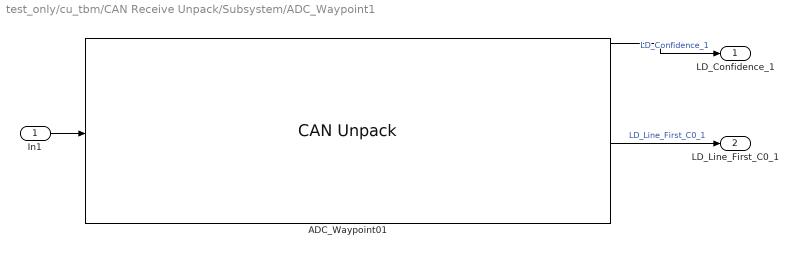
== system test_only/cu_tbm/CAN Receive Unpack/Subsystem/ADC_Waypoint1 ==
  In1 : Inport
  ADC_Waypoint01 : canmsglib/CAN Unpack  CANdbFile=C:\Users\bowen.zheng\Desktop\spdGoat_prj_20230605\spdGoat_prj_20230605\support\dbc\NIO_NT2_Chassis2_CAN_Official_Release_V_1_1_DA_02.dbc  MsgList=ADC1_WayPoint01  MsgName=ADC1_WayPoint01  MsgIDType=Standard (11-bit identifier)  MsgIdentifier=214  MsgLength=8  SignalInfo={'LD_Confidence_1','24','4','BE','unsigned','Standard','0','0.1','0','0','1.5';'LD_First_End_1','51','7','BE','unsigned','Standard','0','1','0','0','127';'LD_First_Start_1','16','8','BE','unsigned','Standard','0','0.1','0','0','25.5';'LD_First_Type_1','28','4','BE','unsigned','Standard','0','1','0','0','15';'LD_Line_First_C0_1','56','11','BE','unsigned','Standard','0','0.01','-10.24','-10.24','10.23';'LD_Line_First_C1_1','43','13','BE','unsigned','Standard','0','0.0001','-0.4096','-0.4096','0.4095';'LD_Line_First_C2_1','0','8','BE','unsigned','Standard','0','0.0001','-0.0128','-0.0128','0.0127';'LD_Line_First_C3_1','8','8','BE','unsigned','Standard','0','1e-06','-0.000128','-0.000128','0.000127'}  IDPort=off  TimestampPort=off  ErrorPort=off  RemotePort=off  LengthPort=off  StatusPort=off  ApplyMinMax=off
      settings: SourceProductBaseCode=ME,VN  DataFormat=CANdb specified signals
  LD_Confidence_1 : Outport
  LD_Line_First_C0_1 : Outport  Port=2
  wires:
  In1/1 -> ADC_Waypoint01/1
  ADC_Waypoint01/1 -> LD_Confidence_1/1  "LD_Confidence_1"
  ADC_Waypoint01/5 -> LD_Line_First_C0_1/1  "LD_Line_First_C0_1"

== system test_only/cu_tbm/CAN Receive Unpack/Subsystem/ADC_Waypoint2 ==
  In1 : Inport
  ADC_Waypoint01 : canmsglib/CAN Unpack  CANdbFile=C:\Users\bowen.zheng\Desktop\spdGoat_prj_20230605\spdGoat_prj_20230605\support\dbc\NIO_NT2_Chassis2_CAN_Official_Release_V_1_1_DA_02.dbc  MsgList=ADC1_WayPoint02  MsgName=ADC1_WayPoint02  MsgIDType=Standard (11-bit identifier)  MsgIdentifier=215  MsgLength=8  SignalInfo={'LD_Confidence_2','24','4','BE','unsigned','Standard','0','0.1','0','0','1.5';'LD_First_End_2','51','7','BE','unsigned','Standard','0','1','0','0','127';'LD_First_Start_2','16','8','BE','unsigned','Standard','0','0.1','0','0','25.5';'LD_First_Type_2','28','4','BE','unsigned','Standard','0','1','0','0','15';'LD_Line_First_C0_2','56','11','BE','unsigned','Standard','0','0.01','-10.24','-10.24','10.23';'LD_Line_First_C1_2','43','13','BE','unsigned','Standard','0','0.0001','-0.4096','-0.4096','0.4095';'LD_Line_First_C2_2','0','8','BE','unsigned','Standard','0','0.0001','-0.0128','-0.0128','0.0127';'LD_Line_First_C3_2','8','8','BE','unsigned','Standard','0','1e-06','-0.000128','-0.000128','0.000127'}  IDPort=off  TimestampPort=off  ErrorPort=off  RemotePort=off  LengthPort=off  StatusPort=off  ApplyMinMax=off
      settings: SourceProductBaseCode=ME,VN  DataFormat=CANdb specified signals
  LD_Confidence_2 : Outport
  LD_Line_First_C0_2 : Outport  Port=2
  wires:
  In1/1 -> ADC_Waypoint01/1
  ADC_Waypoint01/1 -> LD_Confidence_2/1  "LD_Confidence_2"
  ADC_Waypoint01/5 -> LD_Line_First_C0_2/1  "LD_Line_First_C0_2"

== system test_only/cu_tbm/CAN Receive Unpack/Subsystem/ADC_Waypoint3 ==
  In1 : Inport
  ADC_Waypoint01 : canmsglib/CAN Unpack  CANdbFile=C:\Users\bowen.zheng\Desktop\spdGoat_prj_20230605\spdGoat_prj_20230605\support\dbc\NIO_NT2_Chassis2_CAN_Official_Release_V_1_1_DA_02.dbc  MsgList=ADC1_WayPoint03  MsgName=ADC1_WayPoint03  MsgIDType=Standard (11-bit identifier)  MsgIdentifier=216  MsgLength=8  SignalInfo={'LD_Confidence_3','24','4','BE','unsigned','Standard','0','0.1','0','0','1.5';'LD_First_End_3','51','7','BE','unsigned','Standard','0','1','0','0','127';'LD_First_Start_3','16','8','BE','unsigned','Standard','0','0.1','0','0','25.5';'LD_First_Type_3','28','4','BE','unsigned','Standard','0','1','0','0','15';'LD_Line_First_C0_3','56','11','BE','unsigned','Standard','0','0.01','-10.24','-10.24','10.23';'LD_Line_First_C1_3','43','13','BE','unsigned','Standard','0','0.0001','-0.4096','-0.4096','0.4095';'LD_Line_First_C2_3','0','8','BE','unsigned','Standard','0','0.0001','-0.0128','-0.0128','0.0127';'LD_Line_First_C3_3','8','8','BE','unsigned','Standard','0','1e-06','-0.000128','-0.000128','0.000127'}  IDPort=off  TimestampPort=off  ErrorPort=off  RemotePort=off  LengthPort=off  StatusPort=off  ApplyMinMax=off
      settings: SourceProductBaseCode=ME,VN  DataFormat=CANdb specified signals
  LD_Confidence_3 : Outport
  LD_Line_First_C0_3 : Outport  Port=2
  wires:
  In1/1 -> ADC_Waypoint01/1
  ADC_Waypoint01/1 -> LD_Confidence_3/1  "LD_Confidence_3"
  ADC_Waypoint01/5 -> LD_Line_First_C0_3/1  "LD_Line_First_C0_3"

== system test_only/cu_tbm/CAN Receive Unpack/Subsystem/ADC_Waypoint4 ==
  In1 : Inport
  ADC_Waypoint01 : canmsglib/CAN Unpack  CANdbFile=C:\Users\bowen.zheng\Desktop\spdGoat_prj_20230605\spdGoat_prj_20230605\support\dbc\NIO_NT2_Chassis2_CAN_Official_Release_V_1_1_DA_02.dbc  MsgList=ADC1_WayPoint04  MsgName=ADC1_WayPoint04  MsgIDType=Standard (11-bit identifier)  MsgIdentifier=217  MsgLength=8  SignalInfo={'LD_Confidence_4','24','4','BE','unsigned','Standard','0','0.1','0','0','1.5';'LD_First_End_4','51','7','BE','unsigned','Standard','0','1','0','0','127';'LD_First_Start_4','16','8','BE','unsigned','Standard','0','0.1','0','0','25.5';'LD_First_Type_4','28','4','BE','unsigned','Standard','0','1','0','0','15';'LD_Line_First_C0_4','56','11','BE','unsigned','Standard','0','0.01','-10.24','-10.24','10.23';'LD_Line_First_C1_4','43','13','BE','unsigned','Standard','0','0.0001','-0.4096','-0.4096','0.4095';'LD_Line_First_C2_4','0','8','BE','unsigned','Standard','0','0.0001','-0.0128','-0.0128','0.0127';'LD_Line_First_C3_4','8','8','BE','unsigned','Standard','0','1e-06','-0.000128','-0.000128','0.000127'}  IDPort=off  TimestampPort=off  ErrorPort=off  RemotePort=off  LengthPort=off  StatusPort=off  ApplyMinMax=off
      settings: SourceProductBaseCode=ME,VN  DataFormat=CANdb specified signals
  LD_Confidence_4 : Outport
  LD_Line_First_C0_4 : Outport  Port=2
  wires:
  In1/1 -> ADC_Waypoint01/1
  ADC_Waypoint01/1 -> LD_Confidence_4/1  "LD_Confidence_4"
  ADC_Waypoint01/5 -> LD_Line_First_C0_4/1  "LD_Line_First_C0_4"

== matlab function test_only/cu_tbm/Equation/MATLAB Function1 ==
  data: u input; y output
function y = fcn(u)

 y = 0.01 * u - 6.04;

== matlab function test_only/cu_tbm/Equation/MATLAB Function2 ==
  data: u input; y output
function y = fcn(u)

 y = 0.01 * u - 6.04;

== matlab function test_only/cu_tbm/Equation/MATLAB Function3 ==
  data: u input; y output
function y = fcn(u)

 y = 0.01 * u - 6.04;

== matlab function test_only/cu_tbm/Equation1/MATLAB Function ==
  data: u input; y output
function y = fcn(u)

 y = (u + 6.04) / 0.01;

== matlab function test_only/cu_tbm/Equation1/MATLAB Function1 ==
  data: u input; y output
function y = fcn(u)

 y = (u + 6.04) / 0.01;

== matlab function test_only/cu_tbm/Equation1/MATLAB Function2 ==
  data: u input; y output
function y = fcn(u)

 y = (u + 6.04) / 0.01;

== matlab function test_only/cu_tbm/Equation1/MATLAB Function3 ==
  data: u input; y output
function y = fcn(u)

 y = (u + 6.04) / 0.01;

== matlab function test_only/cu_tbm/write BCU_09/canPack_nt2ch2_v1_1da02.dbc:BCU_09/varabToFixed_8byts ==
  data: u input uint8 size=8; y output uint8
function y = fcn(u)

fixed_size = 8;
y = uint8(zeros(fixed_size,1));

for i=1:fixed_size
    y(i) = u(i);
end

== matlab function test_only/cu_tbm/Equation/MATLAB Function ==
  data: u input; y output
function y = fcn(u)

 y = 0.01 * u - 6.04;
